simulink model "KalmanFilter_Longitudinal"  (R2016b)
settings: Solver=VariableStepAuto  StartTime=0.0  StopTime=100  RelTol=1e-3
undefined symbols (not defined in the file or in its folder): A_long, B_long, C_long, Continuous, D_long, Time
libraries: ctrlSharedLib x1
settings Model: Creator=yashm  LastModifiedBy=yashm

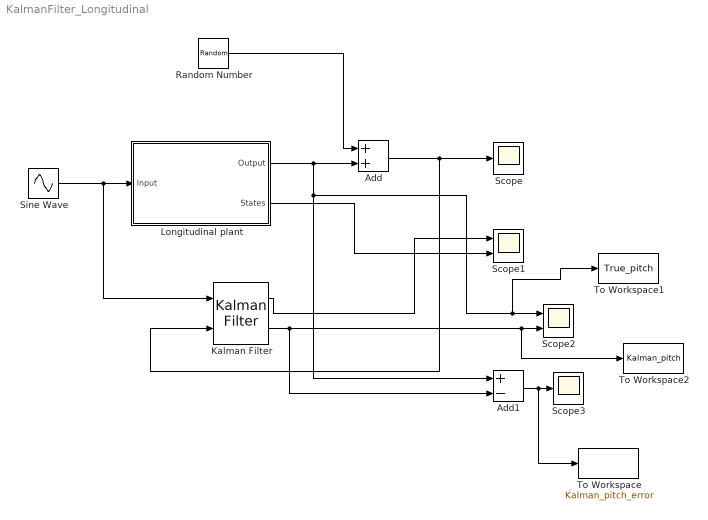
== system KalmanFilter_Longitudinal ==
  Add : Sum
  Add1 : Sum  Inputs=+-
  Kalman Filter : ctrlSharedLib/Kalman Filter  TimeDomain=Continuous-Time  UseCurrentEstimator=on  ModelSource=Individual A, B, C, D matrices  ModelSourceVariable=ss(0.95,1,1,0,1)  A=A_long  B=B_long  C=C_long  D=D_long  NumberOfStates=1  NumberOfInputs=1  NumberOfOutputs=1  InitialEstimateSource=Dialog  X0=0  P0=10  UseK=off  UseGH=off  NumberOfProcessNoiseInputs=1  G=1  TimeInvariantG=on  H=0  TimeInvariantH=on  Q=1  TimeInvariantQ=on  R=1  TimeInvariantR=on  N=0  TimeInvariantN=on  AddInputPort=on  AddEnablePort=off  ExternalReset=none  OutputEstimatedY=on  OutputP=off  Ts=0.01
  Longitudinal plant : Subsystem
  Random Number : RandomNumber  Variance=1e-8  SampleTime=0.01
  Scope : Scope
  Scope1 : Scope  NumInputPorts=2
  Scope2 : Scope  NumInputPorts=2
  Scope3 : Scope
  Sine Wave : Sin  Amplitude=0.1  Frequency=5  SampleTime=0
  To Workspace : ToWorkspace  VariableName=Kalman_pitch_error  SampleTime=0.001
      settings: Save2DSignal=2-D array (concatenate along first dimension)
  To Workspace1 : ToWorkspace  VariableName=True_pitch  SampleTime=0.001
      settings: Save2DSignal=2-D array (concatenate along first dimension)
  To Workspace2 : ToWorkspace  VariableName=Kalman_pitch  SampleTime=0.001
      settings: Save2DSignal=2-D array (concatenate along first dimension)
  wires:
  Sine Wave/1 -> Kalman Filter/1, Longitudinal plant/1(Input)
  Random Number/1 -> Add/1
  Kalman Filter/1 -> Scope1/1
  Add/1 -> Kalman Filter/2, Scope/1
  Longitudinal plant/2(States) -> Scope1/2
  Kalman Filter/2 -> Add1/2, To Workspace2/1, Scope2/2
  Longitudinal plant/1(Output) -> Add1/1, Scope2/1, To Workspace1/1, Add/2
  Add1/1 -> To Workspace/1, Scope3/1

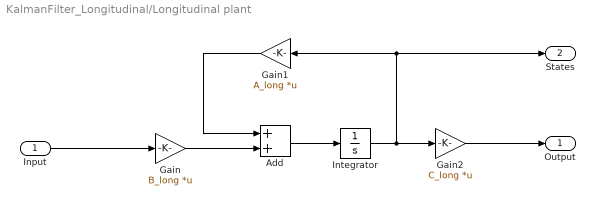
== system KalmanFilter_Longitudinal/Longitudinal plant ==
  Input : Inport
  Add : Sum
  Gain : Gain  Gain=B_long  Multiplication=Matrix(K*u)
  Gain1 : Gain  Gain=A_long  Multiplication=Matrix(K*u)
  Gain2 : Gain  Gain=C_long  Multiplication=Matrix(K*u)
  Integrator : Integrator
  Output : Outport
  States : Outport  Port=2
  wires:
  Gain2/1 -> Output/1
  Input/1 -> Gain/1
  Gain/1 -> Add/2
  Integrator/1 -> Gain1/1, States/1, Gain2/1
  Add/1 -> Integrator/1
  Gain1/1 -> Add/1
